simulink library "INT_AirCtl_Gov"  (R2016b)
settings: Solver=VariableStepAuto  StartTime=0.0  StopTime=10.0  RelTol=1e-3
settings Model: Creator=zhulinfeng  LastModifiedBy=zhulinfeng

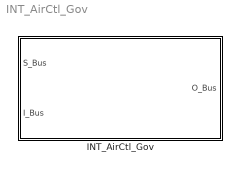
== system INT_AirCtl_Gov ==
  INT_AirCtl_Gov : Subsystem

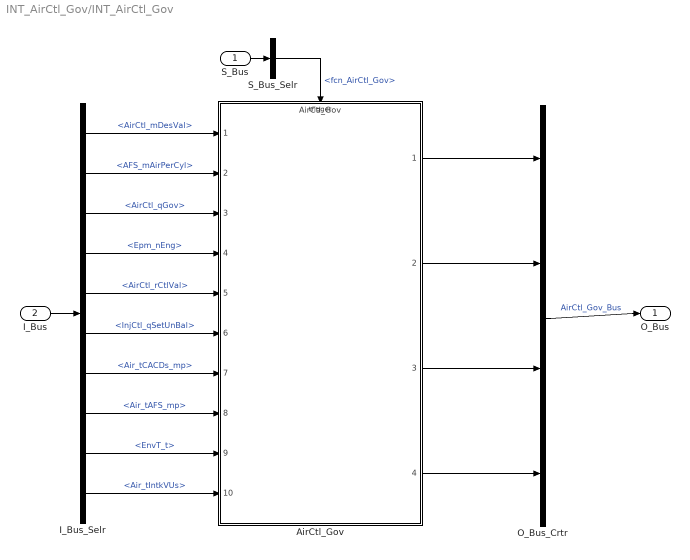
== system INT_AirCtl_Gov/INT_AirCtl_Gov ==
  S_Bus : Inport
  I_Bus : Inport  Port=2
  AirCtl_Gov : ModelReference  ModelNameDialog=AirCtl_Gov  SimulationMode=Normal  ModelReferenceVersion=1.100  TriggerPortName=function  TriggerPortTriggerType=function-call  TriggerPortStatesWhenEnabling=held
  I_Bus_Selr : BusSelector  OutputSignals=AirCtl_mDesVal,AFS_mAirPerCyl,AirCtl_qGov,Epm_nEng,AirCtl_rCtlVal,InjCtl_qSetUnBal,Air_tCACDs_mp,Air_tAFS_mp,EnvT_t,Air_tIntkVUs
  O_Bus_Crtr : BusCreator  Inputs=4
  S_Bus_Selr : BusSelector  OutputSignals=fcn_AirCtl_Gov
  O_Bus : Outport
  wires:
  S_Bus_Selr/1 -> AirCtl_Gov/Trigger  "<fcn_AirCtl_Gov>"
  S_Bus/1 -> S_Bus_Selr/1
  I_Bus/1 -> I_Bus_Selr/1
  I_Bus_Selr/1 -> AirCtl_Gov/1  "<AirCtl_mDesVal>"
  I_Bus_Selr/2 -> AirCtl_Gov/2  "<AFS_mAirPerCyl>"
  I_Bus_Selr/3 -> AirCtl_Gov/3  "<AirCtl_qGov>"
  I_Bus_Selr/4 -> AirCtl_Gov/4  "<Epm_nEng>"
  I_Bus_Selr/5 -> AirCtl_Gov/5  "<AirCtl_rCtlVal>"
  I_Bus_Selr/6 -> AirCtl_Gov/6  "<InjCtl_qSetUnBal>"
  I_Bus_Selr/7 -> AirCtl_Gov/7  "<Air_tCACDs_mp>"
  I_Bus_Selr/8 -> AirCtl_Gov/8  "<Air_tAFS_mp>"
  I_Bus_Selr/9 -> AirCtl_Gov/9  "<EnvT_t>"
  I_Bus_Selr/10 -> AirCtl_Gov/10  "<Air_tIntkVUs>"
  O_Bus_Crtr/1 -> O_Bus/1  "AirCtl_Gov_Bus"
  AirCtl_Gov/1 -> O_Bus_Crtr/1
  AirCtl_Gov/2 -> O_Bus_Crtr/2
  AirCtl_Gov/3 -> O_Bus_Crtr/3
  AirCtl_Gov/4 -> O_Bus_Crtr/4
